simulink library "templibrary"  (R2020a)
settings: Solver=VariableStepAuto  StartTime=0.0  StopTime=10.0  RelTol=1e-3
undefined symbols (not defined in the file or in its folder): sfunxyauto
settings Model: Creator=seanchai  LastModifiedBy=seanchai
settings DataIOCC: SaveFormat=Array  SignalLoggingSaveFormat=ModelDataLogs  ReturnWorkspaceOutputs=off
settings OptimizationCC: BlockReduction=off  BooleanDataType=off
settings DebuggingCC: SaveWithParameterizedLinksMsg=none  UnderspecifiedInitializationDetection=Classic  MergeDetectMultiDrivingBlocksExec=none  SignalResolutionControl=TryResolveAllWithWarning  MultiTaskDSMMsg=warning  MultiTaskCondExecSysMsg=none
settings HardwareCC: TargetUnknown=on
settings ModelReferenceCC: PropagateSignalLabelsOutOfModel=off
settings ConfigComp: CovMetricSettings=dw  CovHtmlReporting=on

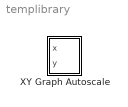
== system templibrary ==
  XY Graph Autoscale : Subsystem  LoadFcn=sfunxyauto([],[],[],'LoadBlock')  StartFcn=sfunxyauto([],[],[],'Start')  StopFcn=sfunxyauto([],[],[],'Stop')  TreatAsAtomicUnit=on  SimViewingDevice=on  mask(XY scope.){xmin=-1, xmax=1, ymin=-1, ymax=1, st=-1}
      mask prompts: xmin "x-min:"; xmax "x-max:"; ymin "y-min:"; ymax "y-max:"; st "Sample time:"
      mask help: XY scope using MATLAB graph window. First input is used as time base. Enter plotting ranges.
      settings: CopyFcn=sfunxyauto([],[],[],'CopyBlock')  DeleteFcn=sfunxyauto([],[],[],'DeleteBlock')  NameChangeFcn=sfunxyauto([],[],[],'NameChange')
      mask Help: This block can be used to explore limit cycles. Look at the m-file sfunxy.m to see how it works.
      mask Display: plot([.05 .95 .95 .05 .05],[.45 .45 .95 .95 .45], 0.5+cos(0:0.1:2*pi)*0.3,0.7+sin(0:0.1:2*pi)*0.2)

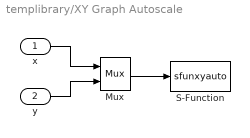
== system templibrary/XY Graph Autoscale ==
  x : Inport
  y : Inport  Port=2
  Mux : Mux  Inputs=2
  S-Function : S-Function  FunctionName=sfunxyauto  Parameters=[xmin xmax ymin ymax], st  SFunctionDeploymentMode=off  EnableBusSupport=off
  wires:
  Mux/1 -> S-Function/1
  x/1 -> Mux/1
  y/1 -> Mux/2
